simulink model "LQR_Model_1_input"  (R2021a)
settings: Solver=FixedStepDiscrete  StartTime=0.0  StopTime=35  FixedStep=1e-3  RelTol=1e-3
values from neighbouring files (symbols this model uses):
  A = []    [Fixed_Model.m]    (also in Matlab_Linear_Model.m = [0 1 ; 0 -Br/I]; Matlab__Linear_Model.m = [0 1 ; 0 Br/I]; Matlab__Linear_Model_2.m = [0 1 ; 0 -Br/I]; Matlab__NonLinear_Model.m = [0 1 ; 0 Br/I])
  B = []    [Fixed_Model.m]    (also in Matlab_Linear_Model.m = [0 ;1]; Matlab__Linear_Model.m = [0 0 ; 1/I -l2x/I]; Matlab__Linear_Model_2.m = [B(:,2)]; Matlab__NonLinear_Model.m = [0 0 ; -H/I -l2x/I])
  C = [1 0]    [Matlab_Linear_Model.m]    (also in Matlab__Linear_Model.m; Matlab__Linear_Model_2.m = [1 1]; Matlab__NonLinear_Model.m; Mc1.mat)
  g = 9.81    [Fixed_Model.m]    (also in Matlab_Linear_Model.m; Matlab__Linear_Model.m; Matlab__Linear_Model_2.m; Matlab__NonLinear_Model.m)
  K = lqr(A,B,Q,R)    [Matlab_Linear_Model.m]    (also in Matlab__Linear_Model.m; Matlab__Linear_Model_2.m; Mc1.mat = [1 0.446480452821]; initialize.m)
  l2f = (l1 + l2)/2 + l3f + l3o    (= 0.65)    [Matlab_Linear_Model.m]    (also in Matlab__Linear_Model_2.m; Mc1.mat; initialize.m; jsp.m)
  l3f = l3o + 0.15    (= 0.3)    [Matlab_Linear_Model.m]    (also in Matlab__Linear_Model.m; Matlab__Linear_Model_2.m; Matlab__NonLinear_Model.m; Mc1.mat)
  l3o = 0.3    [Fixed_Model.m]    (also in Matlab_Linear_Model.m = 0.15; Matlab__Linear_Model.m = 0.15; Matlab__Linear_Model_2.m = 0.15; Matlab__NonLinear_Model.m = 0.15)
  m2 = 2    [Fixed_Model.m]    (also in Matlab_Linear_Model.m = 1.4; Matlab__Linear_Model.m; Matlab__Linear_Model_2.m; Matlab__NonLinear_Model.m = 1.5)
  x0 = [pi/8;0]    [Matlab_Linear_Model.m]    (also in Matlab__Linear_Model.m = [pi/2;0]; Matlab__Linear_Model_2.m = [pi/2;0]; Matlab__NonLinear_Model.m = [pi/2;0]; Mc1.mat = [1.57079632679 0])
undefined symbols (not defined in the file or in its folder): DiscIntNeverNeededParam
libraries: simulink x1
settings Model: Creator=DANI-TUF  LastModifiedBy=DANI-TUF
settings OptimizationCC: DefaultParameterBehavior=Inlined  UseDivisionForNetSlopeComputation=on  GainParamInheritBuiltInType=on  UseFloatMulNetSlope=on  InlineInvariantSignals=on  EnhancedBackFolding=on  BooleansAsBitfields=on  PassReuseOutputArgsAs=Individual arguments  StateBitsets=on  DataBitsets=on  ZeroExternalMemoryAtStartup=off  ZeroInternalMemoryAtStartup=off  NoFixptDivByZeroProtection=on  EfficientFloat2IntCast=on  LifeSpan=1  OptimizeBlockOrder=speed  DifferentSizesBufferReuse=on  EfficientTunableParamExpr=on
settings DebuggingCC: ParameterTunabilityLossMsg=error  SFUnexpectedBacktrackingDiag=warning  SFNoUnconditionalDefaultTransitionDiag=warning
settings HardwareCC: ProdBitPerPointer=32  ProdBitPerSizeT=32  ProdBitPerPtrDiffT=32  ProdLargestAtomicInteger=Long  ProdLargestAtomicFloat=Double  ProdWordSize=32  ProdHWDeviceType=ARM Compatible->ARM Cortex-A
settings SFSimCC: MATLABDynamicMemAlloc=off
settings RTWCC: SystemTargetFile=ert.tlc  TemplateMakefile=ert_default_tmf  GenerateReport=on  BuildConfiguration=Debug  LaunchReport=on  TargetLang=C++
settings CodeAppCC: ForceParamTrailComments=on  IgnoreCustomStorageClasses=off  OperatorAnnotations=on  SimulinkDataObjDesc=on  SFDataObjDesc=on  CustomSymbolStrGlobalVar=rt$N$M  CustomSymbolStrType=$N$M  CustomSymbolStrFcn=$N$M$F  CustomSymbolStrMacro=$N$M  InsertBlockDesc=on  EnableCustomComments=on
settings ERTTargetCC: TargetLangStandard=C++03 (ISO)  GenerateSampleERTMain=on  IncludeMdlTerminateFcn=off  CombineSignalStateStructs=on  CodeInterfacePackaging=C++ class  SupportComplex=off  SupportContinuousTime=on  InlinedParameterPlacement=NonHierarchical  RootIOFormat=Structure reference  ERTCustomFileTemplate=example_file_process.tlc  ERTFilePackagingFormat=CompactWithDataFile

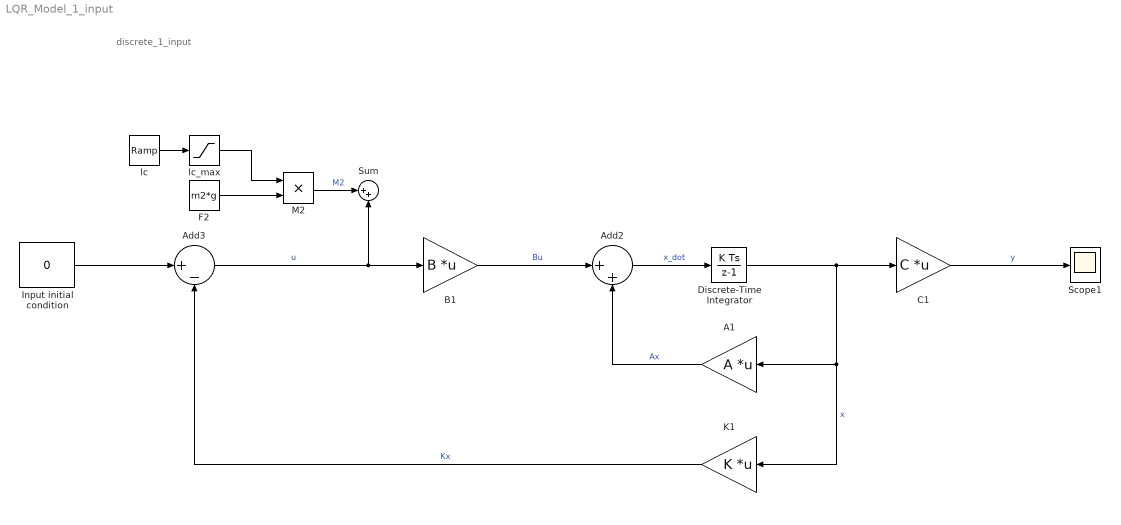
== system LQR_Model_1_input ==
  note: discrete_1_input
  A1 : Gain  Gain=A  Multiplication=Matrix(K*u)
  Add2 : Sum  Inputs=|++
  Add3 : Sum  Inputs=|+-
  B1 : Gain  Gain=B  Multiplication=Matrix(K*u)
  C1 : Gain  Gain=C  Multiplication=Matrix(K*u)
  Discrete-Time Integrator : DiscreteIntegrator  InitialCondition=x0  SampleTime=1e-3  ICPrevOutput=DiscIntNeverNeededParam  ICPrevScaledInput=DiscIntNeverNeededParam
  F2 : Constant  Value=m2*g
  Input initial condition : Constant  Value=0
  K1 : Gain  Gain=K  Multiplication=Matrix(K*u)
  M2 : Product
  Scope1 : Scope
  Sum : Sum  Inputs=|++
  lc : simulink/Sources/Ramp  slope=0.025  start=15  InitialOutput=l2f+l3o-l3f
  lc_max : Saturate  UpperLimit=l2f
  wires:
  C1/1 -> Scope1/1  "y"
  A1/1 -> Add2/2  "Ax"
  Input initial condition/1 -> Add3/1
  B1/1 -> Add2/1  "Bu"
  Discrete-Time Integrator/1 -> C1/1, K1/1, A1/1  "x"
  Add2/1 -> Discrete-Time Integrator/1  "x_dot"
  K1/1 -> Add3/2  "Kx"
  Add3/1 -> B1/1, Sum/2  "u"
  F2/1 -> M2/2
  lc/1 -> lc_max/1
  lc_max/1 -> M2/1
  M2/1 -> Sum/1  "M2"
